simulink subsystem "timeDomainFeatures"  (R2020b)
settings: Solver=VariableStepAuto  StartTime=0.0  StopTime=10.0  RelTol=1e-3
settings Model: Creator=trevvvy  LastModifiedBy=trevor
settings DebuggingCC: SFMachineParentedDataDiag=error

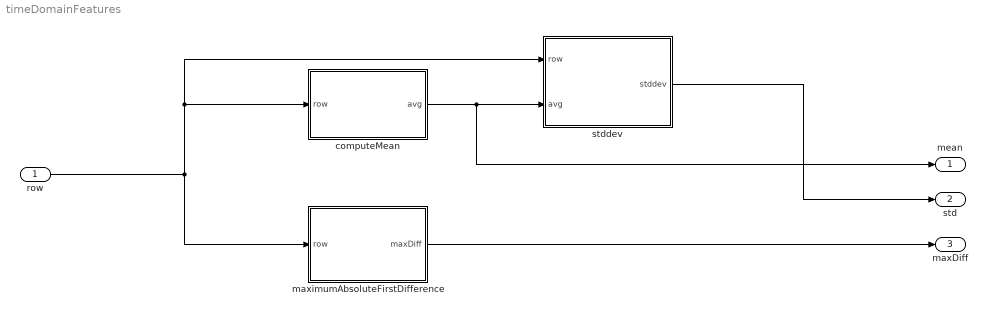
== system timeDomainFeatures ==
  row : Inport  OutMin=0  OutMax=1
  computeMean : Subsystem
  maximumAbsoluteFirstDifference : Subsystem
  stddev : Subsystem
  mean : Outport
  std : Outport  Port=2
  maxDiff : Outport  Port=3
  wires:
  row/1 -> stddev/1(row), computeMean/1(row), maximumAbsoluteFirstDifference/1(row)
  computeMean/1(avg) -> mean/1, stddev/2(avg)
  maximumAbsoluteFirstDifference/1(maxDiff) -> maxDiff/1
  stddev/1(stddev) -> std/1

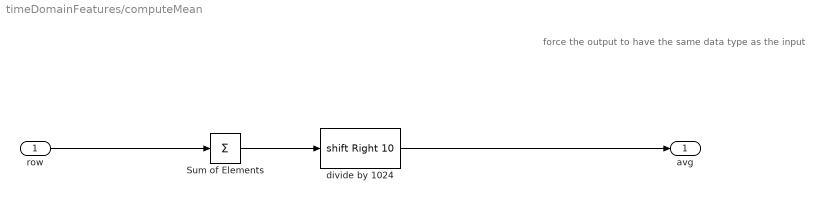
== system timeDomainFeatures/computeMean ==
  note: force the output to have the same data type as the input
  row : Inport
  Sum of Elements : Sum  Inputs=+
  divide by 1024 : ArithShift  BitShiftNumber=10  BitShiftDirection=Right
  avg : Outport
  wires:
  row/1 -> Sum of Elements/1
  Sum of Elements/1 -> divide by 1024/1
  divide by 1024/1 -> avg/1

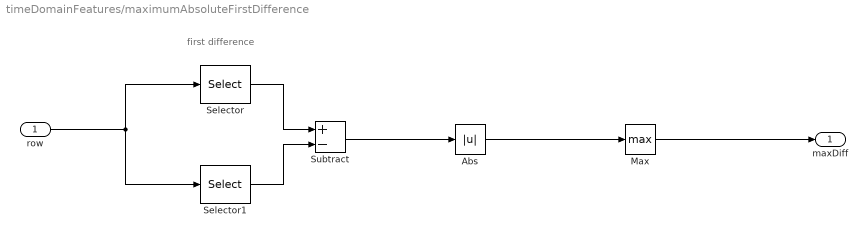
== system timeDomainFeatures/maximumAbsoluteFirstDifference ==
  note: first difference
  row : Inport
  Abs : Abs  OutDataTypeStr=Inherit: Inherit via internal rule
  Max : MinMax  Function=max
  Selector : Selector  InputPortWidth=1024  IndexOptions=Index vector (dialog)  Indices=[2:1024]  OutputSizes=1
  Selector1 : Selector  InputPortWidth=1024  IndexOptions=Index vector (dialog)  Indices=[1:1023]  OutputSizes=1
  Subtract : Sum  Inputs=+-
  maxDiff : Outport
  wires:
  Max/1 -> maxDiff/1
  Subtract/1 -> Abs/1
  row/1 -> Selector1/1, Selector/1
  Abs/1 -> Max/1
  Selector/1 -> Subtract/1
  Selector1/1 -> Subtract/2

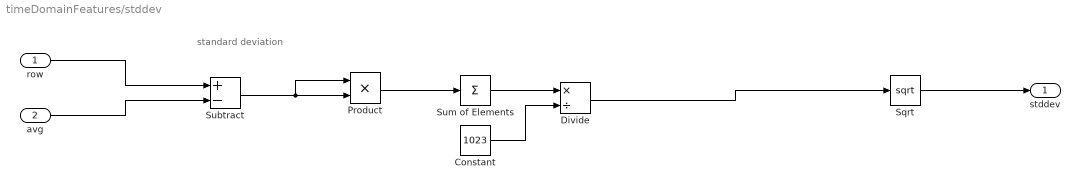
== system timeDomainFeatures/stddev ==
  note: standard deviation
  row : Inport
  avg : Inport  Port=2
  Constant : Constant  Value=1023  OutDataTypeStr=Inherit: Inherit via back propagation  SampleTime=-1
  Divide : Product  Inputs=*/  RndMeth=Simplest  SaturateOnIntegerOverflow=on
  Product : Product
  Sqrt : Sqrt  SaturateOnIntegerOverflow=on
  Subtract : Sum  Inputs=+-
  Sum of Elements : Sum  Inputs=+
  stddev : Outport
  wires:
  Sum of Elements/1 -> Divide/1
  row/1 -> Subtract/1
  Sqrt/1 -> stddev/1
  Subtract/1 -> Product/2, Product/1
  avg/1 -> Subtract/2
  Product/1 -> Sum of Elements/1
  Divide/1 -> Sqrt/1
  Constant/1 -> Divide/2
